simulink model "w2"  (R2020b)
settings: Solver=ode3  StartTime=0.0  StopTime=0.1  FixedStep=1/44100  MaxStep=0.0001  RelTol=1e-3
libraries: powerlib x1
settings Model: Creator=雨后星空  LastModifiedBy=雨后星空
settings DataIOCC: ReturnWorkspaceOutputs=off

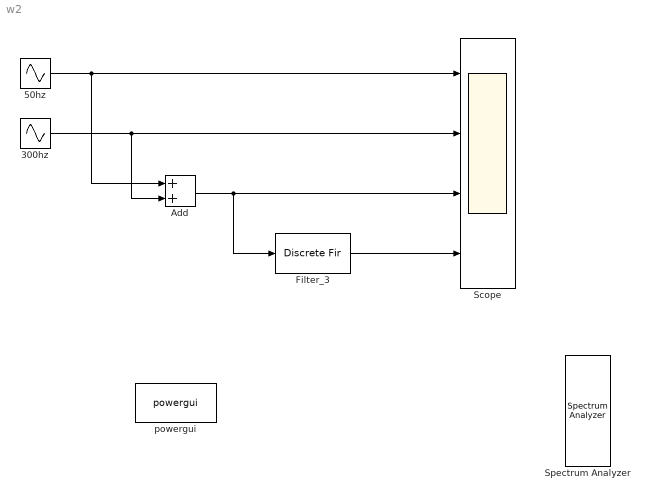
== system w2 ==
  300hz : Sin  Amplitude=100  Frequency=300*2*pi  SampleTime=0
  50hz : Sin  Amplitude=100  Frequency=50*2*pi  SampleTime=0
  Add : Sum
  Filter_3 : DiscreteFir  Tag=BlockMethodSubSystem  Coefficients=[-0.000367126694754497755 -0.00036594039566067402 -0.000364900058315522746 -0.000364003894192419604 -0.000363250041389006771 -0.000362636565256048025 -0.000362161459048927997 -0.00036182264460161268 -0.000361617973022879396 -0.000361545225414607453 -0.000361602113611928389 -0.000361786280945024631 -0.00036209530302234598 -0.000362526688535029398 -0.000363077880082286948 -0.000363746255017514616 -0.00036452912631489674 -0.000365423743456231448 -0.000366427293337746841 -0.000367536901196621247 -0.000368749631556959429 -0.000370062489194943989 -0.000371472420122877266 -0.000372976312591837521 -0.000374570998112660895 -0.000376253252494945095 -0.000378019796903779511 -0.000379867298933900894 -0.00038179237370095456 -0.000383791584949549436 -0.000385861446177794239 -0.000387998421777969397 -0.000390198928193031082 -0.00039245933508858953 -0.00039477596654003376 -0.000397145102234460162 -0.000399562978687047698 -0.00040202579047153873 -0.00040452969146446109 -0.000407070796102733043 -0.000409645180654286654 -0.000412248884501342544 -0.000414877911435963505 -0.000417528230967510652 -0.000420195779641619382 -0.000422876462370322512 -0.000425566153772924838 -0.000428260699527241819 -0.000430955917730816969 -0.000433647600271715151 -0.000436331514208493148 -0.000439003403158959977 -0.00044165898869729872 -0.000444293971759175525 -0.000446904034054397515 -0.000449484839486728337 -0.000452032035580442128 -0.000454541254913199907 -0.000457008116554837355 -0.000459428227511633779 -0.000461797184175656128 -0.000464110573778746304 -0.000466363975850735471 -0.000468552963681445904 -0.000470673105786082705 -0.000472719967373556773 -0.000474689111817327731 -0.000476576102128350304 -0.000478376502429652816 -0.000480085879432173726 -0.000481699803911375874 -0.00048321385218424019 -0.000484623607586190397 -0.000485924661947524292 -0.00048711261706892167 -0.000488183086195590323 -0.000489131695489624838 -0.000489954085500148863 -0.00049064591263080974 -0.000491202850604187283 -0.000491620591922703356 -0.000491894849325595087 -0.000492021357241521559 -0.000491995873236392763 -0.0004918141794559729 -0.0004914720840628634 -0.000490965422667418426 -0.000490290059752191147 -0.000489441890089476156 -0.000488416840151553234 -0.00048721086951319134 -0.000485819972246023292 -0.000484240178304371036 -0.000482467554902102228 -0.000480498207880148418 -0.000478328283064231429 -0.000475953967612440247 -0.000473371491352247292 -0.000470577128106542428 -0.000467567197008358633 -0.000464338063803815487 -0.000460886142142971687 -0.000457207894858152099 -0.000453299835229407499 -0.00044915852823669306 -0.000444780591798443346 -0.000440162697996123267 -0.000435301574284437034 -0.000430194004686810085 -0.000424836830975775328 -0.000419226953837968002 -0.000413361334023304677 -0.000407236993478074928 -0.000400851016461562231 -0.00039420055064586136 -0.000387282808198607291 -0.000380095066848234412 -0.000372634670931474437 -0.000364899032422792333 -0.000356885631945412594 -0.000348592019763670625 -0.000340015816756371781 -0.000331154715370849154 -0.000322006480557469421 -0.00031256895068426969 -0.000302840038431463762 -0.000292817731665545708 -0.000282500094292718364 -0.000271885267091390213 -0.00026097146852349537 -0.000249756995524367165 -0.000238240224270935505 -0.000226419610928032313 -0.000214293692372524632 -0.000201861086895092044 -0.000189120494879439354 -0.00017607069945867803 -0.000162710567148735384 -0.000149039048458547675 -0.000135055178476870788 -0.000120758077435522863 -0.000106146951248842821 -9.12210920292587656e-05 -7.5979878578732985e-05 -6.04227768559843724e-05 -4.45493404192841481e-05 -2.83592108447160768e-05 -1.1852118119751257e-05 4.97211898798613244e-06 2.21135925869068618e-05 3.95723053426901174e-05 5.73481701846755294e-05 7.54410100375605433e-05 9.38505575783965713e-05 0.000112576455019107761 0.00013161825391449586 0.000150975414995859993 0.000170647308030314967 0.000190633211705809868 0.000210932313541953135 0.000231543709826657077 ...(+12733 chars)]  InputProcessing=Columns as channels (frame based)
  Scope : Scope  NumInputPorts=4
  Spectrum Analyzer : SpectrumAnalyzer  NumInputPorts=4
  powergui : powerlib/powergui  Priority=1  SimulationMode=Continuous  SampleTime=50e-6  frequency=60  Iterations=50  frequencyindice=60  Pbase=100e6  ErrMax=1e-4  UnitsV=kV  UnitsW=MW  buscounter=0  FunctionMessages=off  echomessages=off  EnableUseOfTLC=off  CurrentSourceSwitches=off  DisableSnubberDevices=off  DisableRonSwitches=off  DisableVfSwitches=off  DisplayEquations=off  AutomaticDiscreteSolvers=off  SolverType=Tustin/Backward Euler (TBE)  Interpol=off  ExternalGateDelay=off  methode=off  Ts=100  x0status=blocks  SPID=on  SwTol=0  HookPort=off  NonlinearTolerance=1e-4  nMaxIteration=100  ContinueOnMaxIteration=off  RestoreLinks=warning  ResistiveCurrentMeasurement=off  Frange=[0:2:500]  Ylog=off  Xlog=on  ShowGrid=off  save=off  variable=ZData  structure=ScopeData  ZoomFFT=off  StartTime=0.02  cycles=1  DisplayStyle=1  fundamental=50  FreqAxis=off  MaxFrequency=100  frequencyindicesteady=1  RmsSteady=1  display=off
  wires:
  Add/1 -> Filter_3/1, Scope/3
  50hz/1 -> Add/1, Scope/1
  300hz/1 -> Add/2, Scope/2
  Filter_3/1 -> Scope/4
